simulink model "StateAction_vs_ConditionAction"  (R2018b)
settings: Solver=FixedStepDiscrete  StartTime=0.0  StopTime=10.0  RelTol=1e-3
libraries: simulink x1
settings Model: Creator=marwan  LastModifiedBy=marwan

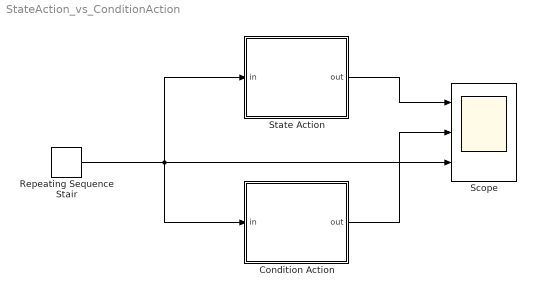
== system StateAction_vs_ConditionAction ==
  Condition Action : Stateflow chart  TreatAsAtomicUnit=on
  Repeating Sequence Stair : simulink/Sources/Repeating Sequence Stair  OutValues=[0 3 6 4 2 7 6]  tsamp=-1  OutMin=[]  OutMax=[]  OutDataTypeStr=double  OutputDataTypeScalingMode=double  OutDataType=fixdt(0,8)  ConRadixGroup=Best Precision: Vector-wise  OutScaling=2^-12
  Scope : Scope  NumInputPorts=3
  State Action : Stateflow chart  TreatAsAtomicUnit=on
  wires:
  State Action/1(out) -> Scope/1
  Condition Action/1(out) -> Scope/2
  Repeating Sequence Stair/1 -> State Action/1(in), Scope/3, Condition Action/1(in)

== stateflow chart StateAction_vs_ConditionAction/Condition Action ==
  state State1
  state State2
  State1 -> State2 : [in>5]{out=2;}
  (default) -> State1
  State2 -> State1 : [in<=5]{out=1;}
  data: in input; out output

== stateflow chart StateAction_vs_ConditionAction/State Action ==
  state State1
    en: out=1;
  state State2
    en: out=2;
  State1 -> State2 : [in>5]
  (default) -> State1
  State2 -> State1 : [in<=5]
  data: in input; out output
